simulink model "Project_1"  (R2023b)
settings: Solver=ode1  StartTime=0.0  StopTime=25  FixedStep=0.1  RelTol=1e-3
values from neighbouring files (symbols this model uses):
  A = 1    [Project1Week2.m]    (also in ProjectWeek1.m; Project_1.m = 4)
  b = 1    [Project1Week2.m]    (also in ProjectWeek1.m; Project_1.m)
  J = 1    [Project1Week2.m]    (also in ProjectWeek1.m; Project_1.m)
  w_0 = 1    [Project1Week2.m]    (also in ProjectWeek1.m; Project_1.m)
settings Model: Creator=Julian Tan  LastModifiedBy=Julian Tan

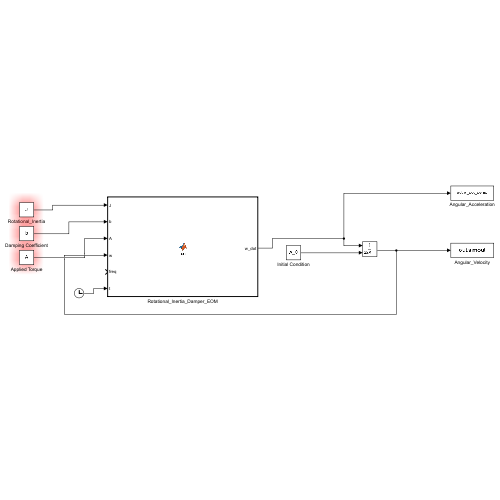
[thumbnail: Simulink's stored preview of the top-level diagram]
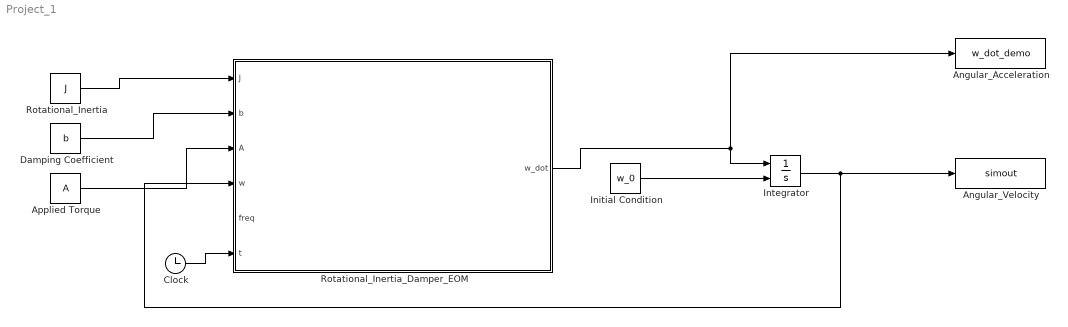
== system Project_1 ==
  Angular_Acceleration : ToWorkspace  VariableName=w_dot_demo  SaveFormat=Timeseries  SampleTime=-1
  Angular_Velocity : ToWorkspace  VariableName=simout  SaveFormat=Timeseries  SampleTime=-1
  Applied Torque : Constant  Value=A
  Clock : Clock
  Damping Coefficient : Constant  Value=b
  Initial Condition : Constant  Value=w_0
  Integrator : Integrator  InitialConditionSource=external
  Rotational_Inertia : Constant  Value=J
  Rotational_Inertia_Damper_EOM : MATLAB Function  TreatAsAtomicUnit=on
  wires:
  Rotational_Inertia/1 -> Rotational_Inertia_Damper_EOM/1(J)
  Damping Coefficient/1 -> Rotational_Inertia_Damper_EOM/2(b)
  Applied Torque/1 -> Rotational_Inertia_Damper_EOM/3(A)
  Rotational_Inertia_Damper_EOM/1(w_dot) -> Angular_Acceleration/1, Integrator/1
  Initial Condition/1 -> Integrator/2
  Integrator/1 -> Angular_Velocity/1, Rotational_Inertia_Damper_EOM/4(w)
  Clock/1 -> Rotational_Inertia_Damper_EOM/6(t)

== matlab function Project_1/Rotational_Inertia_Damper_EOM ==
  data: J input; w_dot output; b input; A input; w input; freq input; t input
function w_dot = fcn(J, b, A, w, freq, t)

w_dot = (1/J)*(A-b*w);


end
